simulink library "INT_AirSys_Lib"  (R2016b)
settings: Solver=VariableStepAuto  StartTime=0.0  StopTime=10.0  RelTol=1e-3
settings Model: Creator=GaberXu  LastModifiedBy=GaberXu

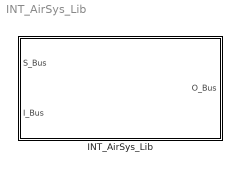
== system INT_AirSys_Lib ==
  INT_AirSys_Lib : Subsystem

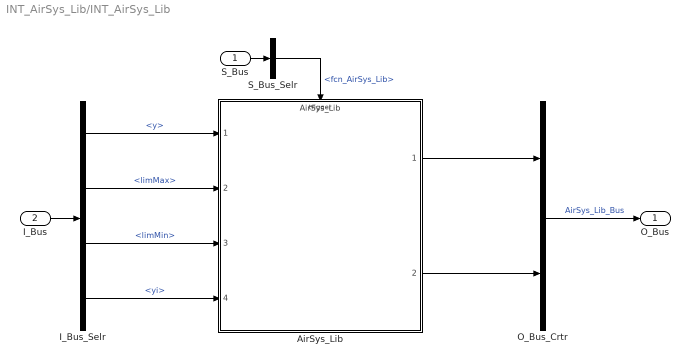
== system INT_AirSys_Lib/INT_AirSys_Lib ==
  S_Bus : Inport
  I_Bus : Inport  Port=2
  AirSys_Lib : ModelReference  ModelNameDialog=AirSys_Lib  ModelReferenceVersion=1.7  TriggerPortName=function  TriggerPortTriggerType=function-call  TriggerPortStatesWhenEnabling=held
  I_Bus_Selr : BusSelector  OutputSignals=y,limMax,limMin,yi
  O_Bus_Crtr : BusCreator  Inputs=2
  S_Bus_Selr : BusSelector  OutputSignals=fcn_AirSys_Lib
  O_Bus : Outport
  wires:
  S_Bus_Selr/1 -> AirSys_Lib/Trigger  "<fcn_AirSys_Lib>"
  S_Bus/1 -> S_Bus_Selr/1
  I_Bus/1 -> I_Bus_Selr/1
  I_Bus_Selr/1 -> AirSys_Lib/1  "<y>"
  I_Bus_Selr/2 -> AirSys_Lib/2  "<limMax>"
  I_Bus_Selr/3 -> AirSys_Lib/3  "<limMin>"
  I_Bus_Selr/4 -> AirSys_Lib/4  "<yi>"
  O_Bus_Crtr/1 -> O_Bus/1  "AirSys_Lib_Bus"
  AirSys_Lib/1 -> O_Bus_Crtr/1
  AirSys_Lib/2 -> O_Bus_Crtr/2
